simulink library "Lib_Vol_Volume_TMATS"  (R2015a)
settings: Solver=ode45  StartTime=0.0  StopTime=10.0  RelTol=1e-3
undefined symbols (not defined in the file): Fluid
libraries: Lib_Vol_PropLookup_TMATS x1
Description:
  | Thomas Modules
settings Model: Creator=jwchapm2  LastModifiedBy=jwchapm2
settings OptimizationCC: ExpressionDepthLimit=2147483647
settings DebuggingCC: UnderspecifiedInitializationDetection=Classic  MergeDetectMultiDrivingBlocksExec=none  SolverPrmCheckMsg=warning  StateNameClashWarn=warning

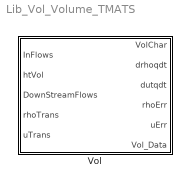
== system Lib_Vol_Volume_TMATS ==
  Vol : Subsystem  mask(T-MATS: Volume Library Block){volume_M=1, htVec_M=Fluid.Vec.ht, PtVec_M=Fluid.Vec.Pt, TtArray_M=Fluid.Array.Tt, uArray_M=Fluid.Array.u, rhoArray_M=Fluid.Array.rho}
      mask prompts: volume_M "volume_M - Volume [in3]"; htVec_M "htVec_M - enthalpy Vector"; PtVec_M "PtVec_M - Pressure Vector"; TtArray_M "TtArray_M - Total Temparture Array f(ht,Pt)"; uArray_M "uArray_M - interal energy Array f(ht,Pt)"; rhoArray_M "rhoArray_M - density Array f(ht,Pt)"
      mask help: This block simulates the performance of a Volume summing all incoming and outgoing flows then computing convergence criteria based on density and internal energy of the flows.
      mask Help: web(which('Vol_TMATS_Vol.html'),'-helpbrowser')

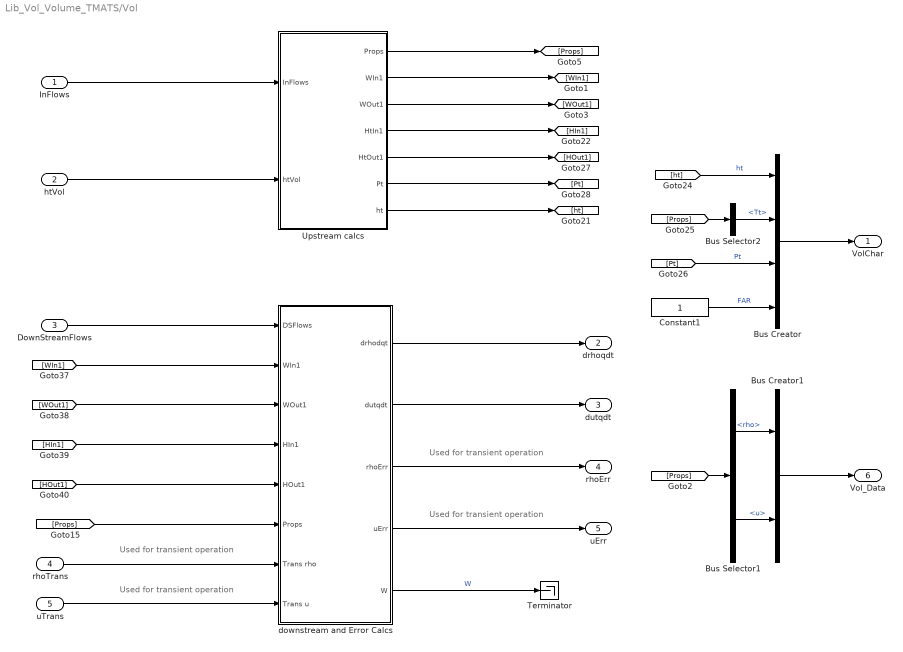
== system Lib_Vol_Volume_TMATS/Vol ==
  note: Used for transient operation
  note: Used for transient operation
  note: Used for transient operation
  note: Used for transient operation
  InFlows : Inport
  htVol : Inport  Port=2
  DownStreamFlows : Inport  Port=3
  rhoTrans : Inport  Port=4
  uTrans : Inport  Port=5
  Bus Creator : BusCreator
  Bus Creator1 : BusCreator  Inputs=2
  Bus Selector1 : BusSelector  OutputSignals=rho,u
  Bus Selector2 : BusSelector  OutputSignals=Tt
  Constant1 : Constant
  Terminator : Terminator
  Upstream calcs : Subsystem  TreatAsAtomicUnit=on
  downstream and Error Calcs : Subsystem  TreatAsAtomicUnit=on
  VolChar : Outport  PortDimensions=4
  drhoqdt : Outport  Port=2  PortDimensions=1
  dutqdt : Outport  Port=3  PortDimensions=1
  rhoErr : Outport  Port=4  PortDimensions=1
  uErr : Outport  Port=5  PortDimensions=1
  Vol_Data : Outport  Port=6  PortDimensions=2
  wires:
  htVol/1 -> Upstream calcs/2(htVol)
  Upstream calcs/1(Props) -> [Props]
  Upstream calcs/2(WIn1) -> [WIn1]
  Upstream calcs/3(WOut1) -> [WOut1]
  Upstream calcs/4(HtIn1) -> [HIn1]
  Upstream calcs/5(HtOut1) -> [HOut1]
  Upstream calcs/6(Pt) -> [Pt]
  DownStreamFlows/1 -> downstream and Error Calcs/1(DSFlows)
  [WIn1] -> downstream and Error Calcs/2(WIn1)
  [WOut1] -> downstream and Error Calcs/3(WOut1)
  [HIn1] -> downstream and Error Calcs/4(HIn1)
  [HOut1] -> downstream and Error Calcs/5(HOut1)
  [Props] -> downstream and Error Calcs/6(Props)
  rhoTrans/1 -> downstream and Error Calcs/7(Trans rho)
  uTrans/1 -> downstream and Error Calcs/8(Trans u)
  downstream and Error Calcs/1(drhodqt) -> drhoqdt/1
  downstream and Error Calcs/2(dutqdt) -> dutqdt/1
  downstream and Error Calcs/3(rhoErr) -> rhoErr/1
  downstream and Error Calcs/4(uErr) -> uErr/1
  Bus Creator/1 -> VolChar/1
  [ht] -> Bus Creator/1  "ht"
  [Props] -> Bus Selector2/1
  Bus Selector2/1 -> Bus Creator/2  "<Tt>"
  [Pt] -> Bus Creator/3  "Pt"
  Upstream calcs/7(ht) -> [ht]
  Constant1/1 -> Bus Creator/4  "FAR"
  downstream and Error Calcs/5(W) -> Terminator/1  "W"
  InFlows/1 -> Upstream calcs/1(InFlows)
  [Props] -> Bus Selector1/1
  Bus Selector1/1 -> Bus Creator1/1  "<rho>"
  Bus Selector1/2 -> Bus Creator1/2  "<u>"
  Bus Creator1/1 -> Vol_Data/1

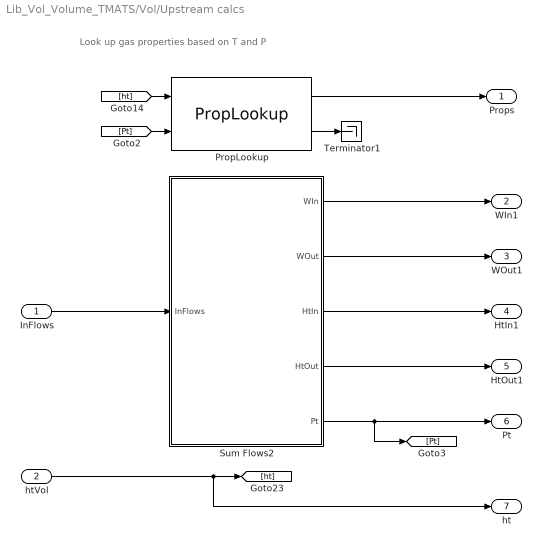
== system Lib_Vol_Volume_TMATS/Vol/Upstream calcs ==
  note: Look up gas properties based on T and P
  InFlows : Inport
  htVol : Inport  Port=2  PortDimensions=1
  PropLookup : Lib_Vol_PropLookup_TMATS/PropLookup  case_M='ht'  propg_M=0  htg_M=0  htVec_M=htVec_M  PtVec_M=PtVec_M  TtVec_M=[0 10]  sVec_M=[0 10]  htArray_M=ones(2, length(PtVec_M))'  rhoArray_M=rhoArray_M  uArray_M=uArray_M  sArray_M=ones(length(htVec_M), length(PtVec_M))'  muArray_M=ones(length(htVec_M), length(PtVec_M))'  ThArray_M=TtArray_M  CvArray_M=ones(length(htVec_M), length(PtVec_M))'  CpArray_M=ones(length(htVec_M), length(PtVec_M))'  kArray_M=ones(length(htVec_M), length(PtVec_M))'  TsArray_M=ones(2, length(PtVec_M))'  hsArray_M=ones(2, length(PtVec_M))'  Rval_M=0
  Sum Flows2 : MATLAB Function  TreatAsAtomicUnit=on
  Terminator1 : Terminator
  Props : Outport
  WIn1 : Outport  Port=2
  WOut1 : Outport  Port=3
  HtIn1 : Outport  Port=4
  HtOut1 : Outport  Port=5
  Pt : Outport  Port=6
  ht : Outport  Port=7
  wires:
  htVol/1 -> ht/1, [ht]
  PropLookup/1 -> Props/1
  PropLookup/2 -> Terminator1/1
  [Pt] -> PropLookup/2
  [ht] -> PropLookup/1
  InFlows/1 -> Sum Flows2/1(InFlows)
  Sum Flows2/1(WIn) -> WIn1/1
  Sum Flows2/2(WOut) -> WOut1/1
  Sum Flows2/3(HtIn) -> HtIn1/1
  Sum Flows2/4(HtOut) -> HtOut1/1
  Sum Flows2/5(Pt) -> [Pt], Pt/1

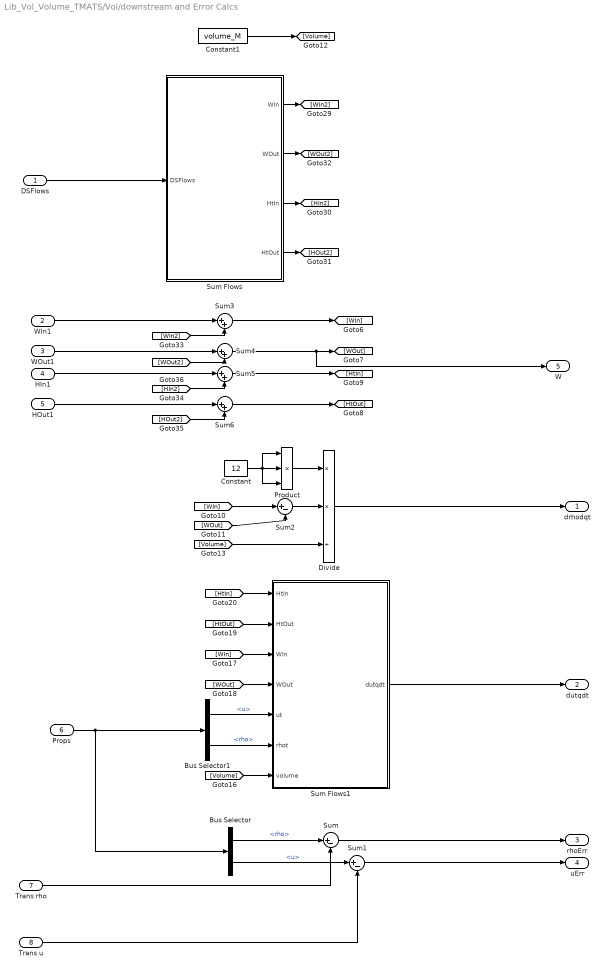
== system Lib_Vol_Volume_TMATS/Vol/downstream and Error Calcs ==
  DSFlows : Inport
  WIn1 : Inport  Port=2
  WOut1 : Inport  Port=3
  HIn1 : Inport  Port=4
  HOut1 : Inport  Port=5
  Props : Inport  Port=6
  Trans rho : Inport  Port=7
  Trans u : Inport  Port=8
  Bus Selector : BusSelector  OutputSignals=rho,u
  Bus Selector1 : BusSelector  OutputSignals=u,rho
  Constant : Constant  Value=12
  Constant1 : Constant  Value=volume_M
  Divide : Product  Inputs=**/
  Product : Product  Inputs=3
  Sum : Sum  Inputs=|+-
  Sum Flows : MATLAB Function  TreatAsAtomicUnit=on
  Sum Flows1 : MATLAB Function  TreatAsAtomicUnit=on
  Sum1 : Sum  Inputs=|+-
  Sum2 : Sum  Inputs=|+-
  Sum{3..6} (4 alike) : Sum  Inputs=|++
  drhodqt : Outport
  dutqdt : Outport  Port=2
  rhoErr : Outport  Port=3
  uErr : Outport  Port=4
  W : Outport  Port=5
  wires:
  Trans rho/1 -> Sum/2
  Trans u/1 -> Sum1/2
  DSFlows/1 -> Sum Flows/1(DSFlows)
  Props/1 -> Bus Selector/1, Bus Selector1/1
  Bus Selector/1 -> Sum/1  "<rho>"
  Bus Selector/2 -> Sum1/1  "<u>"
  [WIn] -> Sum2/1
  [WOut] -> Sum2/2
  Constant/1 -> Product/3, Product/1, Product/2
  Sum2/1 -> Divide/2
  Product/1 -> Divide/1
  [Volume] -> Divide/3
  Constant1/1 -> [Volume]
  Divide/1 -> drhodqt/1
  Bus Selector1/1 -> Sum Flows1/5(ut)  "<u>"
  Bus Selector1/2 -> Sum Flows1/6(rhot)  "<rho>"
  [Volume] -> Sum Flows1/7(volume)
  [WIn] -> Sum Flows1/3(WIn)
  [WOut] -> Sum Flows1/4(WOut)
  [HtOut] -> Sum Flows1/2(HtOut)
  [HtIn] -> Sum Flows1/1(HtIn)
  Sum Flows1/1(dutqdt) -> dutqdt/1
  Sum/1 -> rhoErr/1
  Sum1/1 -> uErr/1
  Sum Flows/1(WIn) -> [WIn2]
  Sum Flows/2(WOut) -> [WOut2]
  Sum Flows/3(HtIn) -> [HIn2]
  Sum Flows/4(HtOut) -> [HOut2]
  WIn1/1 -> Sum3/1
  [WIn2] -> Sum3/2
  WOut1/1 -> Sum4/1
  [WOut2] -> Sum4/2
  Sum4/1 -> W/1, [WOut]
  Sum3/1 -> [WIn]
  HOut1/1 -> Sum6/1
  [HOut2] -> Sum6/2
  [HIn2] -> Sum5/2
  HIn1/1 -> Sum5/1
  Sum5/1 -> [HtIn]
  Sum6/1 -> [HtOut]

== matlab function Lib_Vol_Volume_TMATS/Vol/downstream and Error Calcs/Sum Flows1 ==
  data: HtIn input; HtOut input; WIn input; WOut input; ut input; dutqdt output; rhot input; volume input
function dutqdt = fcn(HtIn,HtOut, WIn, WOut, ut, rhot, volume)
%#codegen

dutqdt = ( HtIn - HtOut - ut * ( WIn - WOut )) / ( rhot * volume/12/12/12 );

== matlab function Lib_Vol_Volume_TMATS/Vol/downstream and Error Calcs/Sum Flows ==
  data: WIn output; WOut output; HtIn output; HtOut output; DSFlows input
function [WIn,WOut, HtIn,HtOut] = fcn(DSFlows)
%#codegen

NumDSFlows = length(DSFlows)/5;

WIn = 0;
WOut = 0;
HtIn = 0;
HtOut = 0;

for i = 1: NumDSFlows
   W = DSFlows((i-1)*5 + 1);
   ht = DSFlows((i-1)*5 + 2);
   if W > 0 
       WOut = WOut + W;
       HtOut = HtOut + W*ht;
   else 
       WIn = WIn - W;
       HtIn = HtIn - W*ht;
   end
end

== matlab function Lib_Vol_Volume_TMATS/Vol/Upstream calcs/Sum Flows2 ==
  data: WIn output; WOut output; HtIn output; HtOut output; Pt output; InFlows input
function [WIn,WOut, HtIn,HtOut, Pt] = fcn(InFlows)
%#codegen

NumInFlows = length(InFlows)/5;

WIn = 0;
WOut = 0;
HtIn = 0;
HtOut = 0;

for i = 1: NumInFlows
   W = InFlows((i-1)*5 + 1);
   ht = InFlows((i-1)*5 + 2);
   if W > 0 
       WIn = WIn + W;
       HtIn = HtIn + W*ht;
   else 
       WOut = WOut - W;
       HtOut = HtOut - W*ht;
   end
end

Pt = InFlows(4);
